simulink model "fiscalnew"  (R2023b)
settings: Solver=VariableStepAuto  StartTime=0.0  StopTime=1.04  RelTol=1e-3
model workspace (MAT data in the model file):
  init_E = 1
values from neighbouring files (symbols this model uses):
  c12 = 0.0008    [fiscal_init.m]    (also in fiscal_tuned.m = 8.2e-05)
  d11 = 0.00005    (= 5e-05)    [fiscal_init.m]    (also in fiscal_tuned.m = 0.0008)
  d12 = -0.000025    (= -2.5e-05)    [fiscal_init.m]    (also in fiscal_tuned.m = -0.0008)
  d13 = 0.0000001    (= 1e-07)    [fiscal_init.m]    (also in fiscal_tuned.m = 1e-05)
  d21 = 0.000015    (= 1.5e-05)    [fiscal_init.m]    (also in fiscal_tuned.m = 0.0001)
  d22 = -0.00001    (= -1e-05)    [fiscal_init.m]    (also in fiscal_tuned.m = -0.0001)
  d23 = 0.00008    (= 8e-05)    [fiscal_init.m]    (also in fiscal_tuned.m = -0.0002)
  t_ef = 0.02    [fiscal_init.m]    (also in fiscal_tuned.m)
  t_if = 0.10    (= 0.1)    [fiscal_init.m]    (also in fiscal_tuned.m)
libraries: simulink x1
settings Model: Creator=olavhegg  LastModifiedBy=olavhegg

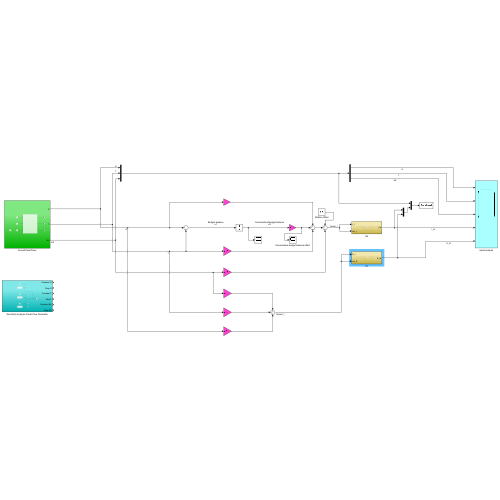
[thumbnail: Simulink's stored preview of the top-level diagram]
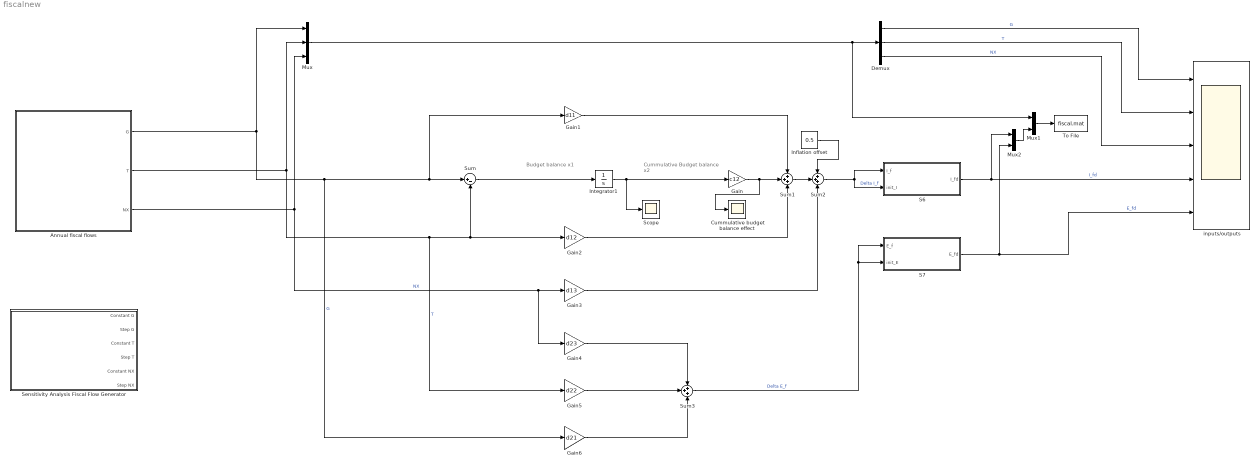
== system fiscalnew ==
  note: Budget balance
      | x1
  note: Cummulative Budget balance
      | x2
  Annual fiscal flows : Subsystem
  Cummulative budget balance effect : Scope
  Demux : Demux  Outputs=3
  Gain : Gain  Gain=c12
  Gain1 : Gain  Gain=d11
  Gain2 : Gain  Gain=d12
  Gain3 : Gain  Gain=d13
  Gain4 : Gain  Gain=d23
  Gain5 : Gain  Gain=d22
  Gain6 : Gain  Gain=d21
  Inflation offset : Constant  Value=0.5
  Integrator1 : Integrator
  Mux : Mux  Inputs=3
  Mux1 : Mux  Inputs=2
  Mux2 : Mux  Inputs=2
  S6 : Subsystem
  S7 : Subsystem
  Scope : Scope
  Sensitivity Analysis Fiscal Flow Generator : Subsystem
  Sum : Sum  Inputs=|+-
  Sum1 : Sum  Inputs=+++
  Sum2 : Sum  Inputs=+++
  Sum3 : Sum  Inputs=+++
  To File : ToFile  Filename=fiscal.mat  MatrixName=fiscalData
  inputs/outputs : Scope  NumInputPorts=5
  wires:
  Sum/1 -> Integrator1/1
  Gain/1 -> Cummulative budget balance effect/1, Sum1/2
  Gain1/1 -> Sum1/1
  Gain2/1 -> Sum1/3
  Sum2/1 -> S6/1(I_f), S6/2(init_I)  "Delta I_f"
  Annual fiscal flows/2(T) -> Gain5/1, Sum/2, Gain2/1, Mux/2  "T"
  Annual fiscal flows/1(G) -> Gain6/1, Gain1/1, Sum/1, Mux/1  "G"
  Sum1/1 -> Sum2/2
  Annual fiscal flows/3(NX) -> Gain4/1, Gain3/1, Mux/3  "NX"
  Gain3/1 -> Sum2/3
  Gain5/1 -> Sum3/2
  Gain4/1 -> Sum3/1
  Gain6/1 -> Sum3/3
  Demux/3 -> inputs/outputs/3  "NX"
  Demux/2 -> inputs/outputs/2  "T"
  Demux/1 -> inputs/outputs/1  "G"
  Integrator1/1 -> Scope/1, Gain/1
  Mux/1 -> Demux/1, Mux1/1
  Mux2/1 -> Mux1/2
  Mux1/1 -> To File/1
  S7/1(E_fd) -> inputs/outputs/5, Mux2/2  "E_fd"
  S6/1(I_fd) -> Mux2/1, inputs/outputs/4  "I_fd"
  Sum3/1 -> S7/1(E_f), S7/2(init_E)  "Delta E_f"
  Inflation offset/1 -> Sum2/1

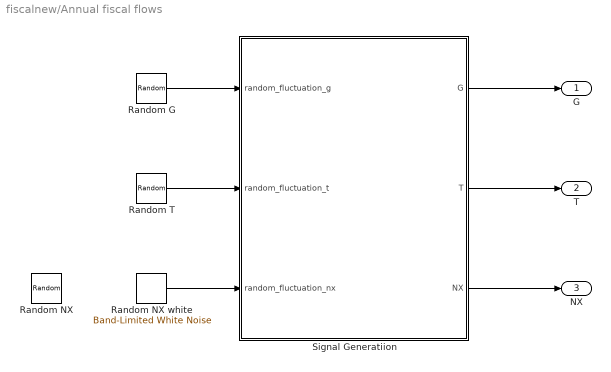
== system fiscalnew/Annual fiscal flows ==
  Random G : RandomNumber  Seed=123  SampleTime=0.12
  Random NX : RandomNumber  Seed=125  SampleTime=0.1
  Random T : RandomNumber  Seed=124  SampleTime=0.12
  Random NX white : simulink/Sources/Band-Limited White Noise  Cov=[0.1]  Ts=0.05  seed=[23341]
  Signal Generatiion : MATLAB Function  TreatAsAtomicUnit=on
  G : Outport
  T : Outport  Port=2
  NX : Outport  Port=3
  wires:
  Signal Generatiion/1(G) -> G/1
  Random T/1 -> Signal Generatiion/2(random_fluctuation_t)
  Random G/1 -> Signal Generatiion/1(random_fluctuation_g)
  Signal Generatiion/2(T) -> T/1
  Random NX white/1 -> Signal Generatiion/3(random_fluctuation_nx)
  Signal Generatiion/3(NX) -> NX/1

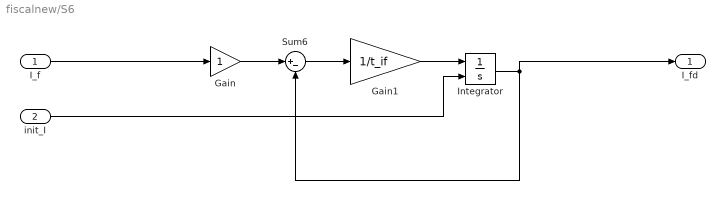
== system fiscalnew/S6 ==
  I_f : Inport
  init_I : Inport  Port=2
  Gain : Gain
  Gain1 : Gain  Gain=1/t_if
  Integrator : Integrator  InitialConditionSource=external
  Sum6 : Sum  Inputs=|+-
  I_fd : Outport
  wires:
  Gain/1 -> Sum6/1
  Gain1/1 -> Integrator/1
  Sum6/1 -> Gain1/1
  I_f/1 -> Gain/1
  Integrator/1 -> I_fd/1, Sum6/2
  init_I/1 -> Integrator/2

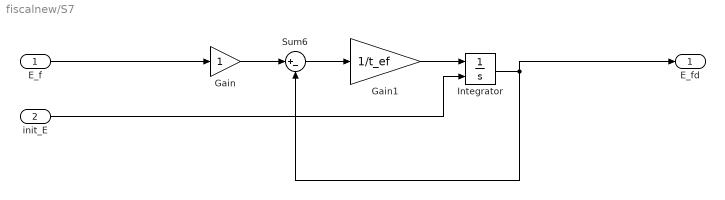
== system fiscalnew/S7 ==
  E_f : Inport
  init_E : Inport  Port=2
  Gain : Gain
  Gain1 : Gain  Gain=1/t_ef
  Integrator : Integrator  InitialConditionSource=external
  Sum6 : Sum  Inputs=|+-
  E_fd : Outport
  wires:
  Gain/1 -> Sum6/1
  Gain1/1 -> Integrator/1
  Sum6/1 -> Gain1/1
  E_f/1 -> Gain/1
  Integrator/1 -> E_fd/1, Sum6/2
  init_E/1 -> Integrator/2

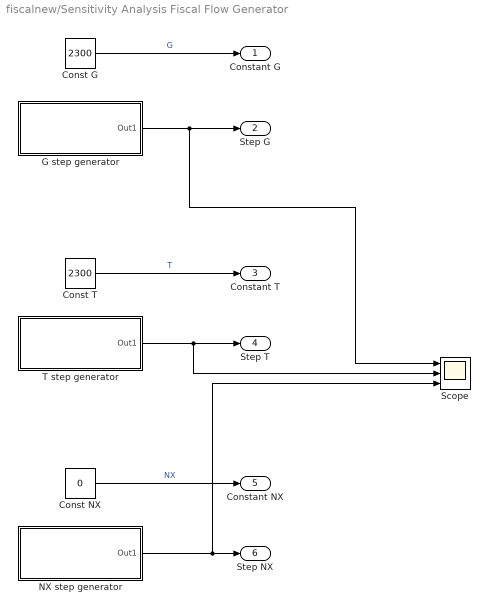
== system fiscalnew/Sensitivity Analysis Fiscal Flow Generator ==
  Const G : Constant  Value=2300
  Const NX : Constant  Value=0
  Const T : Constant  Value=2300
  G step generator : Subsystem
  NX step generator : Subsystem
  Scope : Scope  NumInputPorts=3
  T step generator : Subsystem
  Constant G : Outport
  Step G : Outport  Port=2
  Constant T : Outport  Port=3
  Step T : Outport  Port=4
  Constant NX : Outport  Port=5
  Step NX : Outport  Port=6
  wires:
  Const T/1 -> Constant T/1  "T"
  T step generator/1(Out1) -> Scope/2, Step T/1
  Const NX/1 -> Constant NX/1  "NX"
  NX step generator/1(Out1) -> Scope/3, Step NX/1
  Const G/1 -> Constant G/1  "G"
  G step generator/1(Out1) -> Scope/1, Step G/1

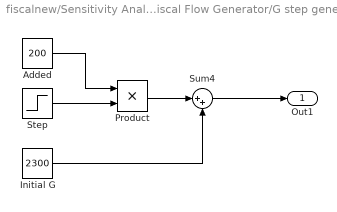
== system fiscalnew/Sensitivity Analysis Fiscal Flow Generator/G step generator ==
  Added : Constant  Value=200
  Initial G : Constant  Value=2300
  Product : Product
  Step : Step  Time=0.10  SampleTime=0
  Sum4 : Sum  Inputs=|++
  Out1 : Outport
  wires:
  Added/1 -> Product/1
  Product/1 -> Sum4/1
  Step/1 -> Product/2
  Initial G/1 -> Sum4/2
  Sum4/1 -> Out1/1

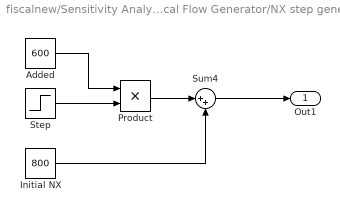
== system fiscalnew/Sensitivity Analysis Fiscal Flow Generator/NX step generator ==
  Added : Constant  Value=600
  Initial NX : Constant  Value=800
  Product : Product
  Step : Step  Time=0.10  SampleTime=0
  Sum4 : Sum  Inputs=|++
  Out1 : Outport
  wires:
  Added/1 -> Product/1
  Product/1 -> Sum4/1
  Step/1 -> Product/2
  Initial NX/1 -> Sum4/2
  Sum4/1 -> Out1/1

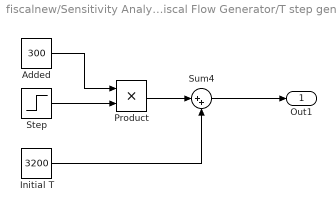
== system fiscalnew/Sensitivity Analysis Fiscal Flow Generator/T step generator ==
  Added : Constant  Value=300
  Initial T : Constant  Value=3200
  Product : Product
  Step : Step  Time=0.10  SampleTime=0
  Sum4 : Sum  Inputs=|++
  Out1 : Outport
  wires:
  Added/1 -> Product/1
  Product/1 -> Sum4/1
  Step/1 -> Product/2
  Initial T/1 -> Sum4/2
  Sum4/1 -> Out1/1

== matlab function fiscalnew/Annual fiscal flows/Signal Generatiion ==
  data: G output; T output; random_fluctuation_g input; random_fluctuation_t input; random_fluctuation_nx input; NX output
function [G, T, NX] = AnnualFiscalFlows(random_fluctuation_g, random_fluctuation_t, random_fluctuation_nx)
    % Constants and initial values (in billion NOK)
    initial_G = 2300;  % Initial government spending in billion NOK
    initial_T = 3200;  % Initial taxation income in billion NOK
    initial_NX = 800;  % Revised average annual net exports in billion NOK

    % Adjusted standard deviation calculation
    max_std_nx = 200;  % Set a maximum standard deviation for NX to 200 billion NOK

    % Variability as a percentage of the initial values
    fluctuation_sensitivity_g = 0.05;  % 5% standard deviation for G
    fluctuation_sensitivity_t = 0.05;  % 5% standard deviation for T
    fluctuation_sensitivity_nx = max_std_nx / initial_NX;  % Use the fixed max std deviation for NX

    % Compute new values for G, T, and NX
    G = initial_G * (1 + fluctuation_sensitivity_g * random_fluctuation_g);
    T = initial_T * (1 + fluctuation_sensitivity_t * random_fluctuation_t);
    NX = initial_NX * (1 + fluctuation_sensitivity_nx * random_fluctuation_nx);
end
